simulink model "s2"  (R2022a)
settings: Solver=VariableStepAuto  StartTime=0.0  StopTime=20  RelTol=1e-6
settings Model: Creator=PC  LastModifiedBy=PC

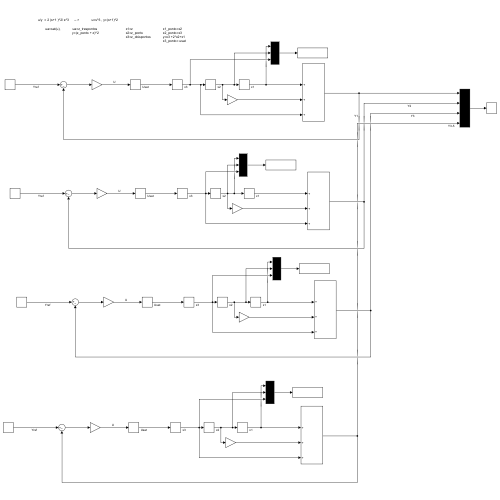
[thumbnail: Simulink's stored preview of the top-level diagram]
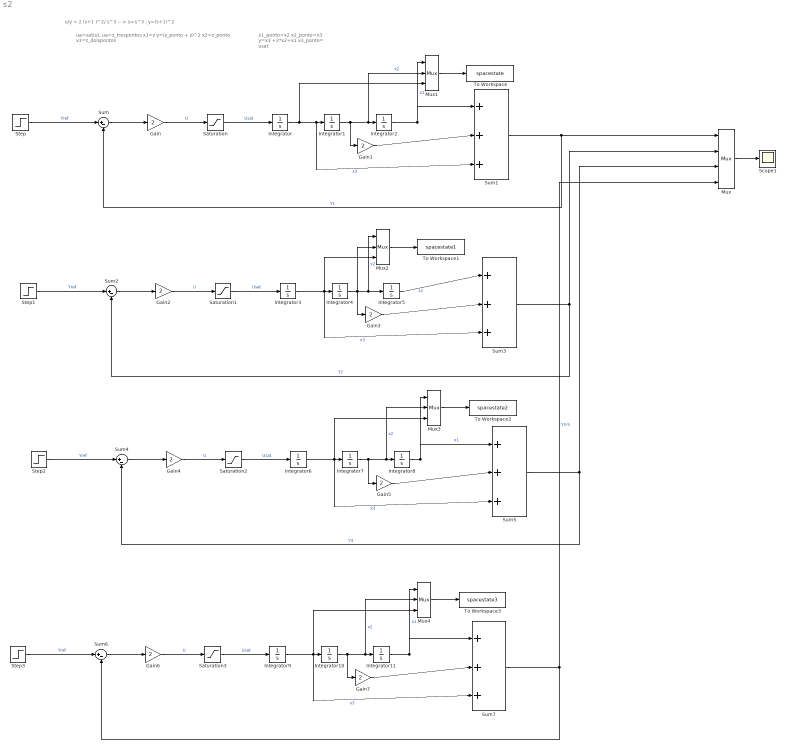
== system s2 ==
  note: x1_ponto=x2
      | x2_ponto=x3
      | y=x3 +2*x2+x1
      | x3_ponto= usat
  note: ua=sat(u),             ua=z_trespontos					x1=z
      | 				y=(z_ponto + z)^2					x2=z_ponto
      | 												x3=z_doispontos
  note: u/y = 2 (s+1 )^2/ s^3 -- > u=s^3 , y=(s+1)^2
  Gain{,1..7} (8 alike) : Gain  Gain=2
  Integrator{,1..11} (12 alike) : Integrator
  Mux : Mux
  Mux{1..4} (4 alike) : Mux  Inputs=3
  Saturation{,1..3} (4 alike) : Saturate  UpperLimit=1  LowerLimit=-1
  Scope1 : Scope
  Step : Step  SampleTime=0
  Step1 : Step  After=2  SampleTime=0
  Step2 : Step  After=3  SampleTime=0
  Step3 : Step  After=3.5  SampleTime=0
  Sum{,2,4,6} (4 alike) : Sum  Inputs=|+-
  Sum{1,3,5,7} (4 alike) : Sum  Inputs=|+++
  To Workspace : ToWorkspace  VariableName=spacestate  SampleTime=-1
  To Workspace1 : ToWorkspace  VariableName=spacestate1  SampleTime=-1
  To Workspace2 : ToWorkspace  VariableName=spacestate2  SampleTime=-1
  To Workspace3 : ToWorkspace  VariableName=spacestate3  SampleTime=-1
  wires:
  Step/1 -> Sum/1  "Yref"
  Sum/1 -> Gain/1
  Gain/1 -> Saturation/1  "U"
  Saturation/1 -> Integrator/1  "Usat"
  Integrator/1 -> Mux1/3, Sum1/3, Integrator1/1  "x3"
  Integrator1/1 -> Gain1/1, Mux1/2, Integrator2/1  "x2"
  Integrator2/1 -> Mux1/1, Sum1/1  "x1"
  Gain1/1 -> Sum1/2
  Sum1/1 -> Sum/2, Mux/1  "Y1"
  Mux/1 -> Scope1/1
  Integrator3/1 -> Sum3/3, Integrator4/1, Mux2/3  "x3"
  Integrator4/1 -> Gain3/1, Mux2/1, Integrator5/1, Mux2/2  "x2"
  Integrator5/1 -> Sum3/1  "x1"
  Sum3/1 -> Mux/2, Sum2/2  "Y2"
  Saturation1/1 -> Integrator3/1  "Usat"
  Gain2/1 -> Saturation1/1  "U"
  Sum2/1 -> Gain2/1
  Step1/1 -> Sum2/1  "Yref"
  Gain3/1 -> Sum3/2
  Integrator6/1 -> Sum5/3, Integrator7/1, Mux3/3  "x3"
  Integrator7/1 -> Gain5/1, Mux3/2, Integrator8/1  "x2"
  Integrator8/1 -> Mux3/1, Sum5/1  "x1"
  Sum5/1 -> Sum4/2, Mux/3  "Y3"
  Saturation2/1 -> Integrator6/1  "Usat"
  Gain4/1 -> Saturation2/1  "U"
  Sum4/1 -> Gain4/1
  Step2/1 -> Sum4/1  "Yref"
  Gain5/1 -> Sum5/2
  Integrator9/1 -> Sum7/3, Integrator10/1, Mux4/3  "x3"
  Integrator10/1 -> Gain7/1, Mux4/2, Integrator11/1  "x2"
  Integrator11/1 -> Mux4/1, Sum7/1  "x1"
  Sum7/1 -> Mux/4, Sum6/2  "Y3-5"
  Saturation3/1 -> Integrator9/1  "Usat"
  Gain6/1 -> Saturation3/1  "U"
  Sum6/1 -> Gain6/1
  Step3/1 -> Sum6/1  "Yref"
  Gain7/1 -> Sum7/2
  Mux1/1 -> To Workspace/1
  Mux2/1 -> To Workspace1/1
  Mux3/1 -> To Workspace2/1
  Mux4/1 -> To Workspace3/1
